simulink model "testModel"  (R2014b)
settings: Solver=ode45  StartTime=0.0  StopTime=10.0  RelTol=1e-3
libraries: simulink x1
settings Model: Creator=YJ_Cao  LastModifiedBy=YJ_Cao

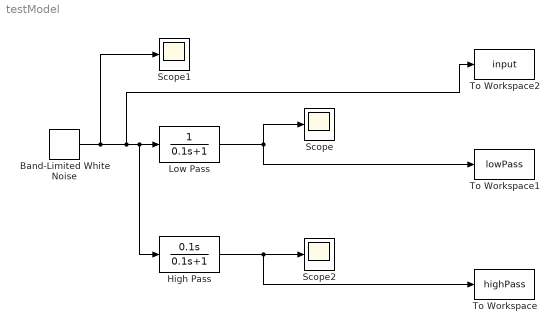
== system testModel ==
  Band-Limited White Noise : simulink/Sources/Band-Limited White Noise  Cov=[0.1]  Ts=0.1  seed=[23341]
  High Pass : TransferFcn  Numerator=[0.1 0]  Denominator=[0.1 1]
  Low Pass : TransferFcn  Denominator=[0.1 1]
  Scope : Scope
  Scope1 : Scope
  Scope2 : Scope
      settings: SaveName=ScopeData2
  To Workspace : ToWorkspace  VariableName=highPass  SaveFormat=Timeseries  SampleTime=-1
  To Workspace1 : ToWorkspace  VariableName=lowPass  SaveFormat=Timeseries  SampleTime=-1
  To Workspace2 : ToWorkspace  VariableName=input  SaveFormat=Timeseries  SampleTime=-1
  wires:
  Band-Limited White Noise/1 -> Scope1/1, To Workspace2/1, High Pass/1, Low Pass/1
  High Pass/1 -> To Workspace/1, Scope2/1
  Low Pass/1 -> Scope/1, To Workspace1/1
